simulink library "inp"  (R2021b)
settings: Solver=VariableStepAuto  StartTime=0.0  StopTime=10.0  RelTol=1e-3
undefined symbols (not defined in the file): C_TASK_5MS_S, FALSE, KINP_AcoreReadyToSlp_flg_ovrdflg, KINP_AcoreReadyToSlp_flg_ovrdval, KINP_AllowMovThd_OTA_enum_ovrdflg, KINP_AllowMovThd_OTA_enum_ovrdval, KINP_APSAngleTarget_Deg_ovrdflg, KINP_APSAngleTarget_Deg_ovrdval, KINP_APSDecReq_mps2_ovrdflg, KINP_APSDecReq_mps2_ovrdval, KINP_APSDecReqA_flg_ovrdflg, KINP_APSDecReqA_flg_ovrdval, KINP_APSDFLL_cm_ovrdflg, KINP_APSDFLL_cm_ovrdval, KINP_APSDFLR_cm_ovrdflg, KINP_APSDFLR_cm_ovrdval, KINP_APSDRLL_cm_ovrdflg, KINP_APSDRLL_cm_ovrdval, KINP_APSDRLR_cm_ovrdflg, KINP_APSDRLR_cm_ovrdval, KINP_APSExitCondition_enum_ovrdflg, KINP_APSExitCondition_enum_ovrdval, KINP_APSHWVer_enum_ovrdflg, KINP_APSHWVer_enum_ovrdval, KINP_APSProgressPCT_pct_ovrdflg, KINP_APSProgressPCT_pct_ovrdval, KINP_APSReq_enum_ovrdflg, KINP_APSReq_enum_ovrdval, KINP_APSRQDisplay_enum_ovrdflg, KINP_APSRQDisplay_enum_ovrdval, KINP_APSRqEPASCtrl_flg_ovrdflg, KINP_APSRqEPASCtrl_flg_ovrdval, KINP_APSShiftPosnReq_enum_ovrdval, KINP_APSShiftPosnReq_enum_ovrflg, KINP_APSSpeedCMD_kph_ovrdval, KINP_APSSpeedCMD_kph_ovrflg, KINP_APSStaSystem_enum_ovrdflg, KINP_APSStaSystem_enum_ovrdval, KINP_APSSWVer_enum_ovrdflg, KINP_APSSWVer_enum_ovrdval, KINP_APSVMCReqA_flg_ovrdval, KINP_APSVMCReqA_flg_ovrflg, KINP_APSVRqEPASCtrl_flg_ovrdflg, KINP_APSVRqEPASCtrl_flg_ovrdval, KINP_AuxBattVolmV_mV_ovrdflg, KINP_AuxBattVolmV_mV_ovrdval, KINP_CAASSta_enum_ovrdflg, KINP_CAASSta_enum_ovrdval, KINP_CAASVMCReqA_flg_ovrdval, KINP_CAASVMCReqA_flg_ovrflg, KINP_Chime_enum_ovrdflg, KINP_Chime_enum_ovrdval, KINP_ClearDTCcmd_flg_ovrdflg, KINP_ClearDTCcmd_flg_ovrdval, KINP_EvccAplusPwrUpReq_flg_ovrdflg, KINP_EvccAplusPwrUpReq_flg_ovrdval, KINP_LFID_raw_ovrdval, KINP_LFID_raw_ovrflg, KINP_LRID_raw_ovrdval, KINP_MemOffsetAccX_raw16_ovrdflg ... (+118)
libraries: FVT_lib x595, hcu_lib x1
(part 25 of 27)

== system inp/INP/CAN4/SignalCheck/Zone_Dr_VCU ==
  BHAL_outputs : Inport
  inp_CanValid_bus : Inport  Port=2
  DrAuBoxPwrN1Curr : FVT_lib/inp/can_signal_template  SystemSampleTime=-1  VariantActivationTime=update diagram  Latency=0  AutoFrameSizeCalculation=off
      link override defval: Value=KINP_DrAuBoxPwrN1Curr_A_defval
      link override fftdec: Value=KINP_DrAuBoxPwrN1Curr_A_fftdec
      link override fftinc: Value=KINP_DrAuBoxPwrN1Curr_A_fftinc
      link override fftlim: Value=KINP_DrAuBoxPwrN1Curr_A_fftlim
      link override invalid: Value=KINP_DrAuBoxPwrN1Curr_A_invalid
      link override ovrdflg: Value=KINP_DrAuBoxPwrN1Curr_A_ovrdflg
      link override ovrdval: Value=KINP_DrAuBoxPwrN1Curr_A_ovrdval
      link override setvalid: Value=KINP_DrAuBoxPwrN1Curr_A_setvalid
      link override srvcflg: Value=KINP_DrAuBoxPwrN1Curr_A_srvcflg
      link override srvcval: Value=KINP_DrAuBoxPwrN1Curr_A_srvcval
  DrAuBoxPwrN2Curr : FVT_lib/inp/can_signal_template  SystemSampleTime=-1  VariantActivationTime=update diagram  Latency=0  AutoFrameSizeCalculation=off
      link override defval: Value=KINP_DrAuBoxPwrN2Curr_A_defval
      link override fftdec: Value=KINP_DrAuBoxPwrN2Curr_A_fftdec
      link override fftinc: Value=KINP_DrAuBoxPwrN2Curr_A_fftinc
      link override fftlim: Value=KINP_DrAuBoxPwrN2Curr_A_fftlim
      link override invalid: Value=KINP_DrAuBoxPwrN2Curr_A_invalid
      link override ovrdflg: Value=KINP_DrAuBoxPwrN2Curr_A_ovrdflg
      link override ovrdval: Value=KINP_DrAuBoxPwrN2Curr_A_ovrdval
      link override setvalid: Value=KINP_DrAuBoxPwrN2Curr_A_setvalid
      link override srvcflg: Value=KINP_DrAuBoxPwrN2Curr_A_srvcflg
      link override srvcval: Value=KINP_DrAuBoxPwrN2Curr_A_srvcval
  DrColumnSWFault : FVT_lib/inp/can_signal_template  SystemSampleTime=-1  VariantActivationTime=update diagram  Latency=0  AutoFrameSizeCalculation=off
      link override defval: Value=KINP_DrColumnSWFault_enum_defval
      link override fftdec: Value=KINP_DrColumnSWFault_enum_fftdec
      link override fftinc: Value=KINP_DrColumnSWFault_enum_fftinc
      link override fftlim: Value=KINP_DrColumnSWFault_enum_fftlim
      link override invalid: Value=KINP_DrColumnSWFault_enum_invalid
      link override ovrdflg: Value=KINP_DrColumnSWFault_enum_ovrdflg
      link override ovrdval: Value=KINP_DrColumnSWFault_enum_ovrdval
      link override setvalid: Value=KINP_DrColumnSWFault_enum_setvalid
      link override srvcflg: Value=KINP_DrColumnSWFault_enum_srvcflg
      link override srvcval: Value=KINP_DrColumnSWFault_enum_srvcval
  DrCtrlBDVolt : FVT_lib/inp/can_signal_template  SystemSampleTime=-1  VariantActivationTime=update diagram  Latency=0  AutoFrameSizeCalculation=off
      link override defval: Value=KINP_DrCtrlBDVolt_V_defval
      link override fftdec: Value=KINP_DrCtrlBDVolt_V_fftdec
      link override fftinc: Value=KINP_DrCtrlBDVolt_V_fftinc
      link override fftlim: Value=KINP_DrCtrlBDVolt_V_fftlim
      link override invalid: Value=KINP_DrCtrlBDVolt_V_invalid
      link override ovrdflg: Value=KINP_DrCtrlBDVolt_V_ovrdflg
      link override ovrdval: Value=KINP_DrCtrlBDVolt_V_ovrdval
      link override setvalid: Value=KINP_DrCtrlBDVolt_V_setvalid
      link override srvcflg: Value=KINP_DrCtrlBDVolt_V_srvcflg
      link override srvcval: Value=KINP_DrCtrlBDVolt_V_srvcval
  DrCtrlTemp : FVT_lib/inp/can_signal_template  SystemSampleTime=-1  VariantActivationTime=update diagram  Latency=0  AutoFrameSizeCalculation=off
      link override defval: Value=KINP_DrCtrlTemp_C_defval
      link override fftdec: Value=KINP_DrCtrlTemp_C_fftdec
      link override fftinc: Value=KINP_DrCtrlTemp_C_fftinc
      link override fftlim: Value=KINP_DrCtrlTemp_C_fftlim
      link override invalid: Value=KINP_DrCtrlTemp_C_invalid
      link override ovrdflg: Value=KINP_DrCtrlTemp_C_ovrdflg
      link override ovrdval: Value=KINP_DrCtrlTemp_C_ovrdval
      link override setvalid: Value=KINP_DrCtrlTemp_C_setvalid
      link override srvcflg: Value=KINP_DrCtrlTemp_C_srvcflg
      link override srvcval: Value=KINP_DrCtrlTemp_C_srvcval
  DrEOBDFault : FVT_lib/inp/can_signal_template  SystemSampleTime=-1  VariantActivationTime=update diagram  Latency=0  AutoFrameSizeCalculation=off
      link override defval: Value=KINP_DrEOBDFault_enum_defval
      link override fftdec: Value=KINP_DrEOBDFault_enum_fftdec
      link override fftinc: Value=KINP_DrEOBDFault_enum_fftinc
      link override fftlim: Value=KINP_DrEOBDFault_enum_fftlim
      link override invalid: Value=KINP_DrEOBDFault_enum_invalid
      link override ovrdflg: Value=KINP_DrEOBDFault_enum_ovrdflg
      link override ovrdval: Value=KINP_DrEOBDFault_enum_ovrdval
      link override setvalid: Value=KINP_DrEOBDFault_enum_setvalid
      link override srvcflg: Value=KINP_DrEOBDFault_enum_srvcflg
      link override srvcval: Value=KINP_DrEOBDFault_enum_srvcval
  DrIVIFault : FVT_lib/inp/can_signal_template  SystemSampleTime=-1  VariantActivationTime=update diagram  Latency=0  AutoFrameSizeCalculation=off
      link override defval: Value=KINP_DrIVIFault_enum_defval
      link override fftdec: Value=KINP_DrIVIFault_enum_fftdec
      link override fftinc: Value=KINP_DrIVIFault_enum_fftinc
      link override fftlim: Value=KINP_DrIVIFault_enum_fftlim
      link override invalid: Value=KINP_DrIVIFault_enum_invalid
      link override ovrdflg: Value=KINP_DrIVIFault_enum_ovrdflg
      link override ovrdval: Value=KINP_DrIVIFault_enum_ovrdval
      link override setvalid: Value=KINP_DrIVIFault_enum_setvalid
      link override srvcflg: Value=KINP_DrIVIFault_enum_srvcflg
      link override srvcval: Value=KINP_DrIVIFault_enum_srvcval
  DrInfoFault : FVT_lib/inp/can_signal_template  SystemSampleTime=-1  VariantActivationTime=update diagram  Latency=0  AutoFrameSizeCalculation=off
      link override defval: Value=KINP_DrInfoFault_enum_defval
      link override fftdec: Value=KINP_DrInfoFault_enum_fftdec
      link override fftinc: Value=KINP_DrInfoFault_enum_fftinc
      link override fftlim: Value=KINP_DrInfoFault_enum_fftlim
      link override invalid: Value=KINP_DrInfoFault_enum_invalid
      link override ovrdflg: Value=KINP_DrInfoFault_enum_ovrdflg
      link override ovrdval: Value=KINP_DrInfoFault_enum_ovrdval
      link override setvalid: Value=KINP_DrInfoFault_enum_setvalid
      link override srvcflg: Value=KINP_DrInfoFault_enum_srvcflg
      link override srvcval: Value=KINP_DrInfoFault_enum_srvcval
  DrPMMLVOutPErrLmp : FVT_lib/inp/can_signal_template  SystemSampleTime=-1  VariantActivationTime=update diagram  Latency=0  AutoFrameSizeCalculation=off
      link override defval: Value=KINP_DrPMMLVOutPErrLmp_flg_defval
      link override fftdec: Value=KINP_DrPMMLVOutPErrLmp_flg_fftdec
      link override fftinc: Value=KINP_DrPMMLVOutPErrLmp_flg_fftinc
      link override fftlim: Value=KINP_DrPMMLVOutPErrLmp_flg_fftlim
      link override invalid: Value=KINP_DrPMMLVOutPErrLmp_flg_invalid
      link override ovrdflg: Value=KINP_DrPMMLVOutPErrLmp_flg_ovrdflg
      link override ovrdval: Value=KINP_DrPMMLVOutPErrLmp_flg_ovrdval
      link override setvalid: Value=KINP_DrPMMLVOutPErrLmp_flg_setvalid
      link override srvcflg: Value=KINP_DrPMMLVOutPErrLmp_flg_srvcflg
      link override srvcval: Value=KINP_DrPMMLVOutPErrLmp_flg_srvcval
  DrPMMLimpHomeActReq : FVT_lib/inp/can_signal_template  SystemSampleTime=-1  VariantActivationTime=update diagram  Latency=0  AutoFrameSizeCalculation=off
      link override defval: Value=KINP_DrPMMLimpHomeActReq_flg_defval
      link override fftdec: Value=KINP_DrPMMLimpHomeActReq_flg_fftdec
      link override fftinc: Value=KINP_DrPMMLimpHomeActReq_flg_fftinc
      link override fftlim: Value=KINP_DrPMMLimpHomeActReq_flg_fftlim
      link override invalid: Value=KINP_DrPMMLimpHomeActReq_flg_invalid
      link override ovrdflg: Value=KINP_DrPMMLimpHomeActReq_flg_ovrdflg
      link override ovrdval: Value=KINP_DrPMMLimpHomeActReq_flg_ovrdval
      link override setvalid: Value=KINP_DrPMMLimpHomeActReq_flg_setvalid
      link override srvcflg: Value=KINP_DrPMMLimpHomeActReq_flg_srvcflg
      link override srvcval: Value=KINP_DrPMMLimpHomeActReq_flg_srvcval
  DrPMMSysErrLmp : FVT_lib/inp/can_signal_template  SystemSampleTime=-1  VariantActivationTime=update diagram  Latency=0  AutoFrameSizeCalculation=off
      link override defval: Value=KINP_DrPMMSysErrLmp_flg_defval
      link override fftdec: Value=KINP_DrPMMSysErrLmp_flg_fftdec
      link override fftinc: Value=KINP_DrPMMSysErrLmp_flg_fftinc
      link override fftlim: Value=KINP_DrPMMSysErrLmp_flg_fftlim
      link override invalid: Value=KINP_DrPMMSysErrLmp_flg_invalid
      link override ovrdflg: Value=KINP_DrPMMSysErrLmp_flg_ovrdflg
      link override ovrdval: Value=KINP_DrPMMSysErrLmp_flg_ovrdval
      link override setvalid: Value=KINP_DrPMMSysErrLmp_flg_setvalid
      link override srvcflg: Value=KINP_DrPMMSysErrLmp_flg_srvcflg
      link override srvcval: Value=KINP_DrPMMSysErrLmp_flg_srvcval
  DrPowerTemp1 : FVT_lib/inp/can_signal_template  SystemSampleTime=-1  VariantActivationTime=update diagram  Latency=0  AutoFrameSizeCalculation=off
      link override defval: Value=KINP_DrPowerTemp1_C_defval
      link override fftdec: Value=KINP_DrPowerTemp1_C_fftdec
      link override fftinc: Value=KINP_DrPowerTemp1_C_fftinc
      link override fftlim: Value=KINP_DrPowerTemp1_C_fftlim
      link override invalid: Value=KINP_DrPowerTemp1_C_invalid
      link override ovrdflg: Value=KINP_DrPowerTemp1_C_ovrdflg
      link override ovrdval: Value=KINP_DrPowerTemp1_C_ovrdval
      link override setvalid: Value=KINP_DrPowerTemp1_C_setvalid
      link override srvcflg: Value=KINP_DrPowerTemp1_C_srvcflg
      link override srvcval: Value=KINP_DrPowerTemp1_C_srvcval
  DrPowerTemp2 : FVT_lib/inp/can_signal_template  SystemSampleTime=-1  VariantActivationTime=update diagram  Latency=0  AutoFrameSizeCalculation=off
      link override defval: Value=KINP_DrPowerTemp2_C_defval
      link override fftdec: Value=KINP_DrPowerTemp2_C_fftdec
      link override fftinc: Value=KINP_DrPowerTemp2_C_fftinc
      link override fftlim: Value=KINP_DrPowerTemp2_C_fftlim
      link override invalid: Value=KINP_DrPowerTemp2_C_invalid
      link override ovrdflg: Value=KINP_DrPowerTemp2_C_ovrdflg
      link override ovrdval: Value=KINP_DrPowerTemp2_C_ovrdval
      link override setvalid: Value=KINP_DrPowerTemp2_C_setvalid
      link override srvcflg: Value=KINP_DrPowerTemp2_C_srvcflg
      link override srvcval: Value=KINP_DrPowerTemp2_C_srvcval
  DrPwrInformationSta : FVT_lib/inp/can_signal_template  SystemSampleTime=-1  VariantActivationTime=update diagram  Latency=0  AutoFrameSizeCalculation=off
      link override defval: Value=KINP_DrPwrInformationSta_flg_defval
      link override fftdec: Value=KINP_DrPwrInformationSta_flg_fftdec
      link override fftinc: Value=KINP_DrPwrInformationSta_flg_fftinc
      link override fftlim: Value=KINP_DrPwrInformationSta_flg_fftlim
      link override invalid: Value=KINP_DrPwrInformationSta_flg_invalid
      link override ovrdflg: Value=KINP_DrPwrInformationSta_flg_ovrdflg
      link override ovrdval: Value=KINP_DrPwrInformationSta_flg_ovrdval
      link override setvalid: Value=KINP_DrPwrInformationSta_flg_setvalid
      link override srvcflg: Value=KINP_DrPwrInformationSta_flg_srvcflg
      link override srvcval: Value=KINP_DrPwrInformationSta_flg_srvcval
  DrPwrONA1Curr : FVT_lib/inp/can_signal_template  SystemSampleTime=-1  VariantActivationTime=update diagram  Latency=0  AutoFrameSizeCalculation=off
      link override defval: Value=KINP_DrPwrONA1Curr_A_defval
      link override fftdec: Value=KINP_DrPwrONA1Curr_A_fftdec
      link override fftinc: Value=KINP_DrPwrONA1Curr_A_fftinc
      link override fftlim: Value=KINP_DrPwrONA1Curr_A_fftlim
      link override invalid: Value=KINP_DrPwrONA1Curr_A_invalid
      link override ovrdflg: Value=KINP_DrPwrONA1Curr_A_ovrdflg
      link override ovrdval: Value=KINP_DrPwrONA1Curr_A_ovrdval
      link override setvalid: Value=KINP_DrPwrONA1Curr_A_setvalid
      link override srvcflg: Value=KINP_DrPwrONA1Curr_A_srvcflg
      link override srvcval: Value=KINP_DrPwrONA1Curr_A_srvcval
  DrPwrONA2Curr : FVT_lib/inp/can_signal_template  SystemSampleTime=-1  VariantActivationTime=update diagram  Latency=0  AutoFrameSizeCalculation=off
      link override defval: Value=KINP_DrPwrONA2Curr_A_defval
      link override fftdec: Value=KINP_DrPwrONA2Curr_A_fftdec
      link override fftinc: Value=KINP_DrPwrONA2Curr_A_fftinc
      link override fftlim: Value=KINP_DrPwrONA2Curr_A_fftlim
      link override invalid: Value=KINP_DrPwrONA2Curr_A_invalid
      link override ovrdflg: Value=KINP_DrPwrONA2Curr_A_ovrdflg
      link override ovrdval: Value=KINP_DrPwrONA2Curr_A_ovrdval
      link override setvalid: Value=KINP_DrPwrONA2Curr_A_setvalid
      link override srvcflg: Value=KINP_DrPwrONA2Curr_A_srvcflg
      link override srvcval: Value=KINP_DrPwrONA2Curr_A_srvcval
  DrPwrSta : FVT_lib/inp/can_signal_template  SystemSampleTime=-1  VariantActivationTime=update diagram  Latency=0  AutoFrameSizeCalculation=off
      link override defval: Value=KINP_DrPwrSta_enum_defval
      link override fftdec: Value=KINP_DrPwrSta_enum_fftdec
      link override fftinc: Value=KINP_DrPwrSta_enum_fftinc
      link override fftlim: Value=KINP_DrPwrSta_enum_fftlim
      link override invalid: Value=KINP_DrPwrSta_enum_invalid
      link override ovrdflg: Value=KINP_DrPwrSta_enum_ovrdflg
      link override ovrdval: Value=KINP_DrPwrSta_enum_ovrdval
      link override setvalid: Value=KINP_DrPwrSta_enum_setvalid
      link override srvcflg: Value=KINP_DrPwrSta_enum_srvcflg
      link override srvcval: Value=KINP_DrPwrSta_enum_srvcval
  DrPwrStdbyACurr : FVT_lib/inp/can_signal_template  SystemSampleTime=-1  VariantActivationTime=update diagram  Latency=0  AutoFrameSizeCalculation=off
      link override defval: Value=KINP_DrPwrStdbyACurr_A_defval
      link override fftdec: Value=KINP_DrPwrStdbyACurr_A_fftdec
      link override fftinc: Value=KINP_DrPwrStdbyACurr_A_fftinc
      link override fftlim: Value=KINP_DrPwrStdbyACurr_A_fftlim
      link override invalid: Value=KINP_DrPwrStdbyACurr_A_invalid
      link override ovrdflg: Value=KINP_DrPwrStdbyACurr_A_ovrdflg
      link override ovrdval: Value=KINP_DrPwrStdbyACurr_A_ovrdval
      link override setvalid: Value=KINP_DrPwrStdbyACurr_A_setvalid
      link override srvcflg: Value=KINP_DrPwrStdbyACurr_A_srvcflg
      link override srvcval: Value=KINP_DrPwrStdbyACurr_A_srvcval
  DrPwrWindowECUFault : FVT_lib/inp/can_signal_template  SystemSampleTime=-1  VariantActivationTime=update diagram  Latency=0  AutoFrameSizeCalculation=off
      link override defval: Value=KINP_DrPwrWindowECUFault_enum_defval
      link override fftdec: Value=KINP_DrPwrWindowECUFault_enum_fftdec
      link override fftinc: Value=KINP_DrPwrWindowECUFault_enum_fftinc
      link override fftlim: Value=KINP_DrPwrWindowECUFault_enum_fftlim
      link override invalid: Value=KINP_DrPwrWindowECUFault_enum_invalid
      link override ovrdflg: Value=KINP_DrPwrWindowECUFault_enum_ovrdflg
      link override ovrdval: Value=KINP_DrPwrWindowECUFault_enum_ovrdval
      link override setvalid: Value=KINP_DrPwrWindowECUFault_enum_setvalid
      link override srvcflg: Value=KINP_DrPwrWindowECUFault_enum_srvcflg
      link override srvcval: Value=KINP_DrPwrWindowECUFault_enum_srvcval
  DrStdAErrSta : FVT_lib/inp/can_signal_template  SystemSampleTime=-1  VariantActivationTime=update diagram  Latency=0  AutoFrameSizeCalculation=off
      link override defval: Value=KINP_DrStdAErrSta_flg_defval
      link override fftdec: Value=KINP_DrStdAErrSta_flg_fftdec
      link override fftinc: Value=KINP_DrStdAErrSta_flg_fftinc
      link override fftlim: Value=KINP_DrStdAErrSta_flg_fftlim
      link override invalid: Value=KINP_DrStdAErrSta_flg_invalid
      link override ovrdflg: Value=KINP_DrStdAErrSta_flg_ovrdflg
      link override ovrdval: Value=KINP_DrStdAErrSta_flg_ovrdval
      link override setvalid: Value=KINP_DrStdAErrSta_flg_setvalid
      link override srvcflg: Value=KINP_DrStdAErrSta_flg_srvcflg
      link override srvcval: Value=KINP_DrStdAErrSta_flg_srvcval
  DrTHCMFault : FVT_lib/inp/can_signal_template  SystemSampleTime=-1  VariantActivationTime=update diagram  Latency=0  AutoFrameSizeCalculation=off
      link override defval: Value=KINP_DrTHCMFault_enum_defval
      link override fftdec: Value=KINP_DrTHCMFault_enum_fftdec
      link override fftinc: Value=KINP_DrTHCMFault_enum_fftinc
      link override fftlim: Value=KINP_DrTHCMFault_enum_fftlim
      link override invalid: Value=KINP_DrTHCMFault_enum_invalid
      link override ovrdflg: Value=KINP_DrTHCMFault_enum_ovrdflg
      link override ovrdval: Value=KINP_DrTHCMFault_enum_ovrdval
      link override setvalid: Value=KINP_DrTHCMFault_enum_setvalid
      link override srvcflg: Value=KINP_DrTHCMFault_enum_srvcflg
      link override srvcval: Value=KINP_DrTHCMFault_enum_srvcval
  Terminator_{1..22} (22 alike) : Terminator
  True_VHAL_DrAuBoxPwrN1Curr_A : Constant  Value=TRUE  OutDataTypeStr=boolean
  True_VHAL_DrAuBoxPwrN2Curr_A : Constant  Value=TRUE  OutDataTypeStr=boolean
  True_VHAL_DrColumnSWFault_enum : Constant  Value=TRUE  OutDataTypeStr=boolean
  True_VHAL_DrCtrlBDVolt_V : Constant  Value=TRUE  OutDataTypeStr=boolean
  True_VHAL_DrCtrlTemp_C : Constant  Value=TRUE  OutDataTypeStr=boolean
  True_VHAL_DrEOBDFault_enum : Constant  Value=TRUE  OutDataTypeStr=boolean
  True_VHAL_DrIVIFault_enum : Constant  Value=TRUE  OutDataTypeStr=boolean
  True_VHAL_DrInfoFault_enum : Constant  Value=TRUE  OutDataTypeStr=boolean
  True_VHAL_DrPMMLVOutPErrLmp_flg : Constant  Value=TRUE  OutDataTypeStr=boolean
  True_VHAL_DrPMMLimpHomeActReq_flg : Constant  Value=TRUE  OutDataTypeStr=boolean
  True_VHAL_DrPMMSysErrLmp_flg : Constant  Value=TRUE  OutDataTypeStr=boolean
  True_VHAL_DrPowerTemp1_C : Constant  Value=TRUE  OutDataTypeStr=boolean
  True_VHAL_DrPowerTemp2_C : Constant  Value=TRUE  OutDataTypeStr=boolean
  True_VHAL_DrPwrInformationSta_flg : Constant  Value=TRUE  OutDataTypeStr=boolean
  True_VHAL_DrPwrONA1Curr_A : Constant  Value=TRUE  OutDataTypeStr=boolean
  True_VHAL_DrPwrONA2Curr_A : Constant  Value=TRUE  OutDataTypeStr=boolean
  True_VHAL_DrPwrSta_enum : Constant  Value=TRUE  OutDataTypeStr=boolean
  True_VHAL_DrPwrStdbyACurr_A : Constant  Value=TRUE  OutDataTypeStr=boolean
  True_VHAL_DrPwrWindowECUFault_enum : Constant  Value=TRUE  OutDataTypeStr=boolean
  True_VHAL_DrStdAErrSta_flg : Constant  Value=TRUE  OutDataTypeStr=boolean
  True_VHAL_DrTHCMFault_enum : Constant  Value=TRUE  OutDataTypeStr=boolean
  True_VHAL_ZoneDrMalfunLevel_enum : Constant  Value=TRUE  OutDataTypeStr=boolean
  ZoneDrMalfunLevel : FVT_lib/inp/can_signal_template  SystemSampleTime=-1  VariantActivationTime=update diagram  Latency=0  AutoFrameSizeCalculation=off
      link override defval: Value=KINP_ZoneDrMalfunLevel_enum_defval
      link override fftdec: Value=KINP_ZoneDrMalfunLevel_enum_fftdec
      link override fftinc: Value=KINP_ZoneDrMalfunLevel_enum_fftinc
      link override fftlim: Value=KINP_ZoneDrMalfunLevel_enum_fftlim
      link override invalid: Value=KINP_ZoneDrMalfunLevel_enum_invalid
      link override ovrdflg: Value=KINP_ZoneDrMalfunLevel_enum_ovrdflg
      link override ovrdval: Value=KINP_ZoneDrMalfunLevel_enum_ovrdval
      link override setvalid: Value=KINP_ZoneDrMalfunLevel_enum_setvalid
      link override srvcflg: Value=KINP_ZoneDrMalfunLevel_enum_srvcflg
      link override srvcval: Value=KINP_ZoneDrMalfunLevel_enum_srvcval
  slr1_{1..22} (22 alike) : BusSelector  OutputSignals=VINP_CANMsgValidZoneDrVCU_flg
  slr_VHAL_DrAuBoxPwrN1Curr_A : BusSelector  OutputSignals=VHAL_DrAuBoxPwrN1Curr_A
  slr_VHAL_DrAuBoxPwrN2Curr_A : BusSelector  OutputSignals=VHAL_DrAuBoxPwrN2Curr_A
  slr_VHAL_DrColumnSWFault_enum : BusSelector  OutputSignals=VHAL_DrColumnSWFault_enum
  slr_VHAL_DrCtrlBDVolt_V : BusSelector  OutputSignals=VHAL_DrCtrlBDVolt_V
  slr_VHAL_DrCtrlTemp_C : BusSelector  OutputSignals=VHAL_DrCtrlTemp_C
  slr_VHAL_DrEOBDFault_enum : BusSelector  OutputSignals=VHAL_DrEOBDFault_enum
  slr_VHAL_DrIVIFault_enum : BusSelector  OutputSignals=VHAL_DrIVIFault_enum
  slr_VHAL_DrInfoFault_enum : BusSelector  OutputSignals=VHAL_DrInfoFault_enum
  slr_VHAL_DrPMMLVOutPErrLmp_flg : BusSelector  OutputSignals=VHAL_DrPMMLVOutPErrLmp_flg
  slr_VHAL_DrPMMLimpHomeActReq_flg : BusSelector  OutputSignals=VHAL_DrPMMLimpHomeActReq_flg
  slr_VHAL_DrPMMSysErrLmp_flg : BusSelector  OutputSignals=VHAL_DrPMMSysErrLmp_flg
  slr_VHAL_DrPowerTemp1_C : BusSelector  OutputSignals=VHAL_DrPowerTemp1_C
  slr_VHAL_DrPowerTemp2_C : BusSelector  OutputSignals=VHAL_DrPowerTemp2_C
  slr_VHAL_DrPwrInformationSta_flg : BusSelector  OutputSignals=VHAL_DrPwrInformationSta_flg
  slr_VHAL_DrPwrONA1Curr_A : BusSelector  OutputSignals=VHAL_DrPwrONA1Curr_A
  slr_VHAL_DrPwrONA2Curr_A : BusSelector  OutputSignals=VHAL_DrPwrONA2Curr_A
  slr_VHAL_DrPwrSta_enum : BusSelector  OutputSignals=VHAL_DrPwrSta_enum
  slr_VHAL_DrPwrStdbyACurr_A : BusSelector  OutputSignals=VHAL_DrPwrStdbyACurr_A
  slr_VHAL_DrPwrWindowECUFault_enum : BusSelector  OutputSignals=VHAL_DrPwrWindowECUFault_enum
  slr_VHAL_DrStdAErrSta_flg : BusSelector  OutputSignals=VHAL_DrStdAErrSta_flg
  slr_VHAL_DrTHCMFault_enum : BusSelector  OutputSignals=VHAL_DrTHCMFault_enum
  slr_VHAL_ZoneDrMalfunLevel_enum : BusSelector  OutputSignals=VHAL_ZoneDrMalfunLevel_enum
  VINP_DrAuBoxPwrN1Curr_A : Outport
  VINP_DrAuBoxPwrN2Curr_A : Outport  Port=2
  VINP_DrColumnSWFault_enum : Outport  Port=3
  VINP_DrCtrlBDVolt_V : Outport  Port=4
  VINP_DrCtrlTemp_C : Outport  Port=5
  VINP_DrEOBDFault_enum : Outport  Port=6
  VINP_DrIVIFault_enum : Outport  Port=7
  VINP_DrInfoFault_enum : Outport  Port=8
  VINP_DrPMMLVOutPErrLmp_flg : Outport  Port=9
  VINP_DrPMMLimpHomeActReq_flg : Outport  Port=10
  VINP_DrPMMSysErrLmp_flg : Outport  Port=11
  VINP_DrPowerTemp1_C : Outport  Port=12
  VINP_DrPowerTemp2_C : Outport  Port=13
  VINP_DrPwrInformationSta_flg : Outport  Port=14
  VINP_DrPwrONA1Curr_A : Outport  Port=15
  VINP_DrPwrONA2Curr_A : Outport  Port=16
  VINP_DrPwrSta_enum : Outport  Port=17
  VINP_DrPwrStdbyACurr_A : Outport  Port=18
  VINP_DrPwrWindowECUFault_enum : Outport  Port=19
  VINP_DrStdAErrSta_flg : Outport  Port=20
  VINP_DrTHCMFault_enum : Outport  Port=21
  VINP_ZoneDrMalfunLevel_enum : Outport  Port=22
  wires:
  BHAL_outputs/1 -> [BHAL_outputs]
  inp_CanValid_bus/1 -> [inp_CanValid_bus]
  [BHAL_outputs] -> slr_VHAL_DrAuBoxPwrN1Curr_A/1
  slr_VHAL_DrAuBoxPwrN1Curr_A/1 -> DrAuBoxPwrN1Curr/1  "<VHAL_DrAuBoxPwrN1Curr_A>"
  True_VHAL_DrAuBoxPwrN1Curr_A/1 -> DrAuBoxPwrN1Curr/2
  [inp_CanValid_bus] -> slr1_1/1
  slr1_1/1 -> DrAuBoxPwrN1Curr/3  "<VINP_CANMsgValidZoneDrVCU_flg>"
  DrAuBoxPwrN1Curr/1 -> VINP_DrAuBoxPwrN1Curr_A/1  "VINP_DrAuBoxPwrN1Curr_A"
  DrAuBoxPwrN1Curr/2 -> Terminator_1/1
  [BHAL_outputs] -> slr_VHAL_DrAuBoxPwrN2Curr_A/1
  slr_VHAL_DrAuBoxPwrN2Curr_A/1 -> DrAuBoxPwrN2Curr/1  "<VHAL_DrAuBoxPwrN2Curr_A>"
  True_VHAL_DrAuBoxPwrN2Curr_A/1 -> DrAuBoxPwrN2Curr/2
  [inp_CanValid_bus] -> slr1_2/1
  slr1_2/1 -> DrAuBoxPwrN2Curr/3  "<VINP_CANMsgValidZoneDrVCU_flg>"
  DrAuBoxPwrN2Curr/1 -> VINP_DrAuBoxPwrN2Curr_A/1  "VINP_DrAuBoxPwrN2Curr_A"
  DrAuBoxPwrN2Curr/2 -> Terminator_2/1
  [BHAL_outputs] -> slr_VHAL_DrColumnSWFault_enum/1
  slr_VHAL_DrColumnSWFault_enum/1 -> DrColumnSWFault/1  "<VHAL_DrColumnSWFault_enum>"
  True_VHAL_DrColumnSWFault_enum/1 -> DrColumnSWFault/2
  [inp_CanValid_bus] -> slr1_3/1
  slr1_3/1 -> DrColumnSWFault/3  "<VINP_CANMsgValidZoneDrVCU_flg>"
  DrColumnSWFault/1 -> VINP_DrColumnSWFault_enum/1  "VINP_DrColumnSWFault_enum"
  DrColumnSWFault/2 -> Terminator_3/1
  [BHAL_outputs] -> slr_VHAL_DrCtrlBDVolt_V/1
  slr_VHAL_DrCtrlBDVolt_V/1 -> DrCtrlBDVolt/1  "<VHAL_DrCtrlBDVolt_V>"
  True_VHAL_DrCtrlBDVolt_V/1 -> DrCtrlBDVolt/2
  [inp_CanValid_bus] -> slr1_4/1
  slr1_4/1 -> DrCtrlBDVolt/3  "<VINP_CANMsgValidZoneDrVCU_flg>"
  DrCtrlBDVolt/1 -> VINP_DrCtrlBDVolt_V/1  "VINP_DrCtrlBDVolt_V"
  DrCtrlBDVolt/2 -> Terminator_4/1
  [BHAL_outputs] -> slr_VHAL_DrCtrlTemp_C/1
  slr_VHAL_DrCtrlTemp_C/1 -> DrCtrlTemp/1  "<VHAL_DrCtrlTemp_C>"
  True_VHAL_DrCtrlTemp_C/1 -> DrCtrlTemp/2
  [inp_CanValid_bus] -> slr1_5/1
  slr1_5/1 -> DrCtrlTemp/3  "<VINP_CANMsgValidZoneDrVCU_flg>"
  DrCtrlTemp/1 -> VINP_DrCtrlTemp_C/1  "VINP_DrCtrlTemp_C"
  DrCtrlTemp/2 -> Terminator_5/1
  [BHAL_outputs] -> slr_VHAL_DrEOBDFault_enum/1
  slr_VHAL_DrEOBDFault_enum/1 -> DrEOBDFault/1  "<VHAL_DrEOBDFault_enum>"
  True_VHAL_DrEOBDFault_enum/1 -> DrEOBDFault/2
  [inp_CanValid_bus] -> slr1_6/1
  slr1_6/1 -> DrEOBDFault/3  "<VINP_CANMsgValidZoneDrVCU_flg>"
  DrEOBDFault/1 -> VINP_DrEOBDFault_enum/1  "VINP_DrEOBDFault_enum"
  DrEOBDFault/2 -> Terminator_6/1
  [BHAL_outputs] -> slr_VHAL_DrIVIFault_enum/1
  slr_VHAL_DrIVIFault_enum/1 -> DrIVIFault/1  "<VHAL_DrIVIFault_enum>"
  True_VHAL_DrIVIFault_enum/1 -> DrIVIFault/2
  [inp_CanValid_bus] -> slr1_7/1
  slr1_7/1 -> DrIVIFault/3  "<VINP_CANMsgValidZoneDrVCU_flg>"
  DrIVIFault/1 -> VINP_DrIVIFault_enum/1  "VINP_DrIVIFault_enum"
  DrIVIFault/2 -> Terminator_7/1
  [BHAL_outputs] -> slr_VHAL_DrInfoFault_enum/1
  slr_VHAL_DrInfoFault_enum/1 -> DrInfoFault/1  "<VHAL_DrInfoFault_enum>"
  True_VHAL_DrInfoFault_enum/1 -> DrInfoFault/2
  [inp_CanValid_bus] -> slr1_8/1
  slr1_8/1 -> DrInfoFault/3  "<VINP_CANMsgValidZoneDrVCU_flg>"
  DrInfoFault/1 -> VINP_DrInfoFault_enum/1  "VINP_DrInfoFault_enum"
  DrInfoFault/2 -> Terminator_8/1
  [BHAL_outputs] -> slr_VHAL_DrPMMLVOutPErrLmp_flg/1
  slr_VHAL_DrPMMLVOutPErrLmp_flg/1 -> DrPMMLVOutPErrLmp/1  "<VHAL_DrPMMLVOutPErrLmp_flg>"
  True_VHAL_DrPMMLVOutPErrLmp_flg/1 -> DrPMMLVOutPErrLmp/2
  [inp_CanValid_bus] -> slr1_9/1
  slr1_9/1 -> DrPMMLVOutPErrLmp/3  "<VINP_CANMsgValidZoneDrVCU_flg>"
  DrPMMLVOutPErrLmp/1 -> VINP_DrPMMLVOutPErrLmp_flg/1  "VINP_DrPMMLVOutPErrLmp_flg"
  DrPMMLVOutPErrLmp/2 -> Terminator_9/1
  [BHAL_outputs] -> slr_VHAL_DrPMMLimpHomeActReq_flg/1
  slr_VHAL_DrPMMLimpHomeActReq_flg/1 -> DrPMMLimpHomeActReq/1  "<VHAL_DrPMMLimpHomeActReq_flg>"
  True_VHAL_DrPMMLimpHomeActReq_flg/1 -> DrPMMLimpHomeActReq/2
  [inp_CanValid_bus] -> slr1_10/1
  slr1_10/1 -> DrPMMLimpHomeActReq/3  "<VINP_CANMsgValidZoneDrVCU_flg>"
  DrPMMLimpHomeActReq/1 -> VINP_DrPMMLimpHomeActReq_flg/1  "VINP_DrPMMLimpHomeActReq_flg"
  DrPMMLimpHomeActReq/2 -> Terminator_10/1
  [BHAL_outputs] -> slr_VHAL_DrPMMSysErrLmp_flg/1
  slr_VHAL_DrPMMSysErrLmp_flg/1 -> DrPMMSysErrLmp/1  "<VHAL_DrPMMSysErrLmp_flg>"
  True_VHAL_DrPMMSysErrLmp_flg/1 -> DrPMMSysErrLmp/2
  [inp_CanValid_bus] -> slr1_11/1
  slr1_11/1 -> DrPMMSysErrLmp/3  "<VINP_CANMsgValidZoneDrVCU_flg>"
  DrPMMSysErrLmp/1 -> VINP_DrPMMSysErrLmp_flg/1  "VINP_DrPMMSysErrLmp_flg"
  DrPMMSysErrLmp/2 -> Terminator_11/1
  [BHAL_outputs] -> slr_VHAL_DrPowerTemp1_C/1
  slr_VHAL_DrPowerTemp1_C/1 -> DrPowerTemp1/1  "<VHAL_DrPowerTemp1_C>"
  True_VHAL_DrPowerTemp1_C/1 -> DrPowerTemp1/2
  [inp_CanValid_bus] -> slr1_12/1
  slr1_12/1 -> DrPowerTemp1/3  "<VINP_CANMsgValidZoneDrVCU_flg>"
  DrPowerTemp1/1 -> VINP_DrPowerTemp1_C/1  "VINP_DrPowerTemp1_C"
  DrPowerTemp1/2 -> Terminator_12/1
  [BHAL_outputs] -> slr_VHAL_DrPowerTemp2_C/1
  slr_VHAL_DrPowerTemp2_C/1 -> DrPowerTemp2/1  "<VHAL_DrPowerTemp2_C>"
  True_VHAL_DrPowerTemp2_C/1 -> DrPowerTemp2/2
  [inp_CanValid_bus] -> slr1_13/1
  slr1_13/1 -> DrPowerTemp2/3  "<VINP_CANMsgValidZoneDrVCU_flg>"
  DrPowerTemp2/1 -> VINP_DrPowerTemp2_C/1  "VINP_DrPowerTemp2_C"
  DrPowerTemp2/2 -> Terminator_13/1
  [BHAL_outputs] -> slr_VHAL_DrPwrInformationSta_flg/1
  slr_VHAL_DrPwrInformationSta_flg/1 -> DrPwrInformationSta/1  "<VHAL_DrPwrInformationSta_flg>"
  True_VHAL_DrPwrInformationSta_flg/1 -> DrPwrInformationSta/2
  [inp_CanValid_bus] -> slr1_14/1
  slr1_14/1 -> DrPwrInformationSta/3  "<VINP_CANMsgValidZoneDrVCU_flg>"
  DrPwrInformationSta/1 -> VINP_DrPwrInformationSta_flg/1  "VINP_DrPwrInformationSta_flg"
  DrPwrInformationSta/2 -> Terminator_14/1
  [BHAL_outputs] -> slr_VHAL_DrPwrONA1Curr_A/1
  slr_VHAL_DrPwrONA1Curr_A/1 -> DrPwrONA1Curr/1  "<VHAL_DrPwrONA1Curr_A>"
  True_VHAL_DrPwrONA1Curr_A/1 -> DrPwrONA1Curr/2
  [inp_CanValid_bus] -> slr1_15/1
  slr1_15/1 -> DrPwrONA1Curr/3  "<VINP_CANMsgValidZoneDrVCU_flg>"
  DrPwrONA1Curr/1 -> VINP_DrPwrONA1Curr_A/1  "VINP_DrPwrONA1Curr_A"
  DrPwrONA1Curr/2 -> Terminator_15/1
  [BHAL_outputs] -> slr_VHAL_DrPwrONA2Curr_A/1
  slr_VHAL_DrPwrONA2Curr_A/1 -> DrPwrONA2Curr/1  "<VHAL_DrPwrONA2Curr_A>"
  True_VHAL_DrPwrONA2Curr_A/1 -> DrPwrONA2Curr/2
  [inp_CanValid_bus] -> slr1_16/1
  slr1_16/1 -> DrPwrONA2Curr/3  "<VINP_CANMsgValidZoneDrVCU_flg>"
  DrPwrONA2Curr/1 -> VINP_DrPwrONA2Curr_A/1  "VINP_DrPwrONA2Curr_A"
  DrPwrONA2Curr/2 -> Terminator_16/1
  [BHAL_outputs] -> slr_VHAL_DrPwrSta_enum/1
  slr_VHAL_DrPwrSta_enum/1 -> DrPwrSta/1  "<VHAL_DrPwrSta_enum>"
  True_VHAL_DrPwrSta_enum/1 -> DrPwrSta/2
  [inp_CanValid_bus] -> slr1_17/1
  slr1_17/1 -> DrPwrSta/3  "<VINP_CANMsgValidZoneDrVCU_flg>"
  DrPwrSta/1 -> VINP_DrPwrSta_enum/1  "VINP_DrPwrSta_enum"
  DrPwrSta/2 -> Terminator_17/1
  [BHAL_outputs] -> slr_VHAL_DrPwrStdbyACurr_A/1
  slr_VHAL_DrPwrStdbyACurr_A/1 -> DrPwrStdbyACurr/1  "<VHAL_DrPwrStdbyACurr_A>"
  True_VHAL_DrPwrStdbyACurr_A/1 -> DrPwrStdbyACurr/2
  [inp_CanValid_bus] -> slr1_18/1
  slr1_18/1 -> DrPwrStdbyACurr/3  "<VINP_CANMsgValidZoneDrVCU_flg>"
  DrPwrStdbyACurr/1 -> VINP_DrPwrStdbyACurr_A/1  "VINP_DrPwrStdbyACurr_A"
  DrPwrStdbyACurr/2 -> Terminator_18/1
  [BHAL_outputs] -> slr_VHAL_DrPwrWindowECUFault_enum/1
  slr_VHAL_DrPwrWindowECUFault_enum/1 -> DrPwrWindowECUFault/1  "<VHAL_DrPwrWindowECUFault_enum>"
  True_VHAL_DrPwrWindowECUFault_enum/1 -> DrPwrWindowECUFault/2
  [inp_CanValid_bus] -> slr1_19/1
  slr1_19/1 -> DrPwrWindowECUFault/3  "<VINP_CANMsgValidZoneDrVCU_flg>"
  DrPwrWindowECUFault/1 -> VINP_DrPwrWindowECUFault_enum/1  "VINP_DrPwrWindowECUFault_enum"
  DrPwrWindowECUFault/2 -> Terminator_19/1
  [BHAL_outputs] -> slr_VHAL_DrStdAErrSta_flg/1
  slr_VHAL_DrStdAErrSta_flg/1 -> DrStdAErrSta/1  "<VHAL_DrStdAErrSta_flg>"
  True_VHAL_DrStdAErrSta_flg/1 -> DrStdAErrSta/2
  [inp_CanValid_bus] -> slr1_20/1
  slr1_20/1 -> DrStdAErrSta/3  "<VINP_CANMsgValidZoneDrVCU_flg>"
  DrStdAErrSta/1 -> VINP_DrStdAErrSta_flg/1  "VINP_DrStdAErrSta_flg"
  DrStdAErrSta/2 -> Terminator_20/1
  [BHAL_outputs] -> slr_VHAL_DrTHCMFault_enum/1
  slr_VHAL_DrTHCMFault_enum/1 -> DrTHCMFault/1  "<VHAL_DrTHCMFault_enum>"
  True_VHAL_DrTHCMFault_enum/1 -> DrTHCMFault/2
  [inp_CanValid_bus] -> slr1_21/1
  slr1_21/1 -> DrTHCMFault/3  "<VINP_CANMsgValidZoneDrVCU_flg>"
  DrTHCMFault/1 -> VINP_DrTHCMFault_enum/1  "VINP_DrTHCMFault_enum"
  DrTHCMFault/2 -> Terminator_21/1
  [BHAL_outputs] -> slr_VHAL_ZoneDrMalfunLevel_enum/1
  slr_VHAL_ZoneDrMalfunLevel_enum/1 -> ZoneDrMalfunLevel/1  "<VHAL_ZoneDrMalfunLevel_enum>"
  True_VHAL_ZoneDrMalfunLevel_enum/1 -> ZoneDrMalfunLevel/2
  [inp_CanValid_bus] -> slr1_22/1
  slr1_22/1 -> ZoneDrMalfunLevel/3  "<VINP_CANMsgValidZoneDrVCU_flg>"
  ZoneDrMalfunLevel/1 -> VINP_ZoneDrMalfunLevel_enum/1  "VINP_ZoneDrMalfunLevel_enum"
  ZoneDrMalfunLevel/2 -> Terminator_22/1
